simulink model "mpc_tgt_calc"  (R2020a)
settings: Solver=ode1  StartTime=0.0  StopTime=2600  FixedStep=0.1  RelTol=1e-3
undefined symbols (not defined in the file): accl, alpha, ang, dist, dt, ideal_point, img_ang, img_dist, kanayama_point, pivot_state, sla_param, slip_point, state, trj_diff, v, w
libraries: simulink x1
settings Model: Creator=nao12  LastModifiedBy=nao12
settings DataIOCC: SaveOutput=off  SignalLogging=off  DSMLogging=off  SaveTime=off  ReturnWorkspaceOutputs=off
settings OptimizationCC: EnhancedBackFolding=on  PassReuseOutputArgsAs=Individual arguments  OptimizeBlockOrder=speed  DifferentSizesBufferReuse=on  OptimizationCustomize=off  EfficientTunableParamExpr=on
settings DebuggingCC: ParameterTunabilityLossMsg=error  ArithmeticOperatorsInVariantConditions=warning
settings SFSimCC: SimCustomHeaderCode="#include \"bus.h\""  SimUserIncludeDirs=../include/  MATLABDynamicMemAlloc=off  CustomCodeUndefinedFunction=UseInterfaceOnly
settings RTWCC: SystemTargetFile=ert.tlc  GenCodeOnly=on  TemplateMakefile=ert_default_tmf  GenerateReport=on  RTWUseSimCustomCode=on  CustomHeaderCode="#include \"bus.h\""  CustomInclude=../include/  IncludeHyperlinkInReport=on  LaunchReport=on  GenerateTraceInfo=on  GenerateTraceReport=on  GenerateTraceReportSl=on  GenerateTraceReportSf=on  GenerateTraceReportEml=on
settings CodeAppCC: GenerateComments=off  IgnoreCustomStorageClasses=off  OperatorAnnotations=on  SimulinkDataObjDesc=on  SFDataObjDesc=on  InsertBlockDesc=on
settings ERTTargetCC: TargetLangStandard=C99 (ISO)  GenerateSampleERTMain=on  SupportAbsoluteTime=off  MultiInstanceERTCode=on  CodeInterfacePackaging=Reusable function  SupportComplex=off  ParenthesesLevel=Minimum  ERTCustomFileTemplate=example_file_process.tlc  EnableUserReplacementTypes=on

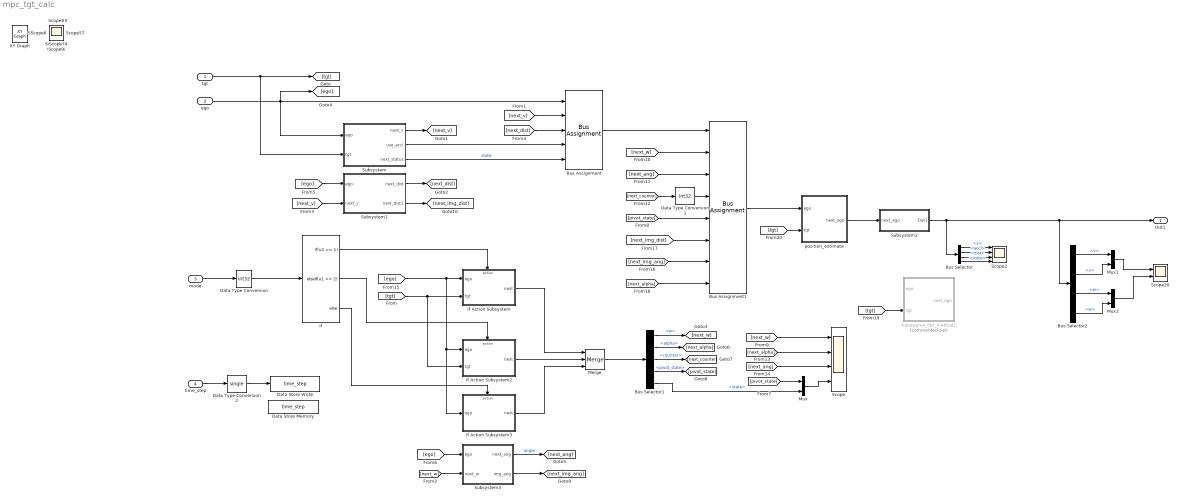
== system mpc_tgt_calc ==
  tgt : Inport  OutDataTypeStr=Bus: t_tgt  BusOutputAsStruct=on
  ego : Inport  Port=2  OutDataTypeStr=Bus: t_ego  BusOutputAsStruct=on
  mode : Inport  Port=3  OutDataTypeStr=int32
  time_step : Inport  Port=4  OutDataTypeStr=int32
  Bus Assignment : BusAssignment  AssignedSignals=v,dist,accl,state
  Bus Assignment1 : BusAssignment  AssignedSignals=w,ang,sla_param.counter,pivot_state,img_dist,img_ang,alpha
  Bus Selector : BusSelector  OutputSignals=v,accl,dist,state
  Bus Selector1 : BusSelector  OutputSignals=w,alpha,sla_param.counter,pivot_state,sla_param.state
  Bus Selector2 : BusSelector  OutputSignals=v,kanayama_point.v,w,kanayama_point.w
  Data Store Memory : DataStoreMemory  DataStoreName=time_step  ReadBeforeWriteMsg=warning  WriteAfterWriteMsg=warning  WriteAfterReadMsg=warning  ShowAdditionalParam=off
  Data Store Write : DataStoreWrite  DataStoreName=time_step
  Data Type Conversion : DataTypeConversion  OutDataTypeStr=int32
  Data Type Conversion1 : DataTypeConversion  OutDataTypeStr=int32
  Data Type Conversion2 : DataTypeConversion  OutDataTypeStr=single
  If : If  IfExpression=u1 == 1  ElseIfExpressions=u1 == 2
  If Action Subsystem : Subsystem  TreatAsAtomicUnit=on
  If Action Subsystem2 : Subsystem  TreatAsAtomicUnit=on
  If Action Subsystem3 : Subsystem  TreatAsAtomicUnit=on
  Merge : Merge  Inputs=3
  Mux : Mux  Inputs=2
  Mux1 : Mux  Inputs=2
  Mux2 : Mux  Inputs=2
  Scope : Scope  NumInputPorts=4
  Scope2 : Scope  NumInputPorts=4
  Scope20 : Scope  NumInputPorts=2
  Subsystem : Subsystem
  Subsystem1 : Subsystem
  Subsystem2 : Subsystem
  Subsystem3 : Subsystem
  kanayama_ctrl_method1 : Subsystem  Commented=on
  position_estimate : Subsystem
  Out1 : Outport  OutDataTypeStr=Bus: t_ego
  Scope{1,3..19} (18 alike) : Scope
  XY Graph : simulink/Sinks/XY Graph  IOType=viewer  xmin=-1  xmax=1  ymin=-1  ymax=1  st=-1
  wires:
  mode/1 -> Data Type Conversion/1
  tgt/1 -> [tgt], Subsystem/2(tgt)
  ego/1 -> Subsystem/1(ego), Bus Assignment/1, [ego]
  Data Type Conversion/1 -> If/1
  If/1 -> If Action Subsystem/Action
  [tgt] -> If Action Subsystem2/2(tgt), If Action Subsystem/2(tgt)
  Bus Assignment/1 -> Bus Assignment1/1
  [next_v] -> Bus Assignment/2
  [next_dist] -> Bus Assignment/3
  Subsystem/1(next_v) -> [next_v]
  [next_v] -> Subsystem1/2(next_v)
  Subsystem1/1(next_dist) -> [next_dist]
  Subsystem/2(use_accl) -> Bus Assignment/4
  Subsystem/3(next_status) -> Bus Assignment/5  "state"
  [next_w] -> Subsystem3/2(next_w)
  [ego] -> Subsystem1/1(ego)
  [ego] -> Subsystem3/1(ego)
  Subsystem3/1(next_ang) -> [next_ang]  "angle"
  Bus Selector/4 -> Scope2/4  "<state>"
  Bus Selector/1 -> Scope2/1  "<v>"
  Bus Selector/2 -> Scope2/2  "<accl>"
  Bus Selector/3 -> Scope2/3  "<dist>"
  Bus Assignment1/1 -> position_estimate/1(ego)
  [next_w] -> Bus Assignment1/2
  [next_ang] -> Bus Assignment1/3
  [next_counter] -> Data Type Conversion1/1
  Data Type Conversion1/1 -> Bus Assignment1/4
  [next_w] -> Scope/1
  [next_alpha] -> Scope/2
  [next_ang] -> Scope/3
  If/2 -> If Action Subsystem2/Action
  [ego] -> If Action Subsystem3/1(ego), If Action Subsystem2/1(ego), If Action Subsystem/1(ego)
  If/3 -> If Action Subsystem3/Action
  Merge/1 -> Bus Selector1/1
  Bus Selector1/1 -> [next_w]  "<w>"
  Bus Selector1/2 -> [next_alpha]  "<alpha>"
  Bus Selector1/3 -> [next_counter]  "<counter>"
  If Action Subsystem/1(next) -> Merge/1
  If Action Subsystem2/1(next) -> Merge/2
  If Action Subsystem3/1(next) -> Merge/3
  Bus Selector1/4 -> [pivot_state]  "<pivot_state>"
  [pivot_state] -> Bus Assignment1/5
  Mux/1 -> Scope/4
  [pivot_state] -> Mux/1
  Bus Selector1/5 -> Mux/2  "<state>"
  Subsystem3/2(img_ang) -> [next_img_ang]
  [next_img_ang] -> Bus Assignment1/7
  Subsystem1/2(next_dist1) -> [next_img_dist]
  [next_img_dist] -> Bus Assignment1/6
  position_estimate/1(next_ego) -> Subsystem2/1(next_ego)
  [next_alpha] -> Bus Assignment1/8
  Subsystem2/1(Out1) -> Bus Selector/1, Out1/1, Bus Selector2/1
  [tgt] -> kanayama_ctrl_method1/2(tgt)
  Mux1/1 -> Scope20/1
  Bus Selector2/1 -> Mux1/1  "<v>"
  Mux2/1 -> Scope20/2
  Bus Selector2/2 -> Mux1/2  "<v>"
  Bus Selector2/3 -> Mux2/1  "<w>"
  Bus Selector2/4 -> Mux2/2  "<w>"
  [tgt] -> position_estimate/2(tgt)
  time_step/1 -> Data Type Conversion2/1
  Data Type Conversion2/1 -> Data Store Write/1

== system mpc_tgt_calc/If Action Subsystem ==
  ego : Inport
  tgt : Inport  Port=2
  Action Port : ActionPort  ActionPortLabel=if(u1 == 1)
  Bus Assignment : BusAssignment  AssignedSignals=w,alpha,sla_param.counter
  Data Type Conversion : DataTypeConversion  OutDataTypeStr=int32
  Data Type Conversion1 : DataTypeConversion  OutDataTypeStr=single
  Data Type Conversion2 : DataTypeConversion  OutDataTypeStr=single
  Subsystem2 : Subsystem
  next : Outport
  wires:
  ego/1 -> Subsystem2/1(ego), Bus Assignment/1
  tgt/1 -> Subsystem2/2(tgt)
  Bus Assignment/1 -> next/1
  Subsystem2/1(next_w) -> Data Type Conversion1/1
  Subsystem2/2(next_alpha) -> Data Type Conversion2/1
  Subsystem2/3(next_count) -> Data Type Conversion/1
  Data Type Conversion/1 -> Bus Assignment/4
  Data Type Conversion1/1 -> Bus Assignment/2
  Data Type Conversion2/1 -> Bus Assignment/3

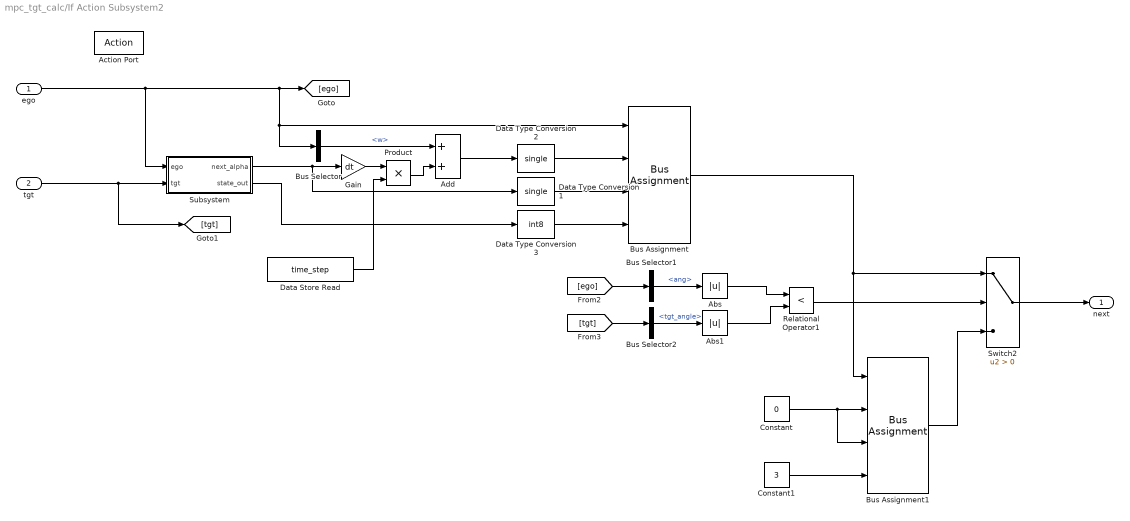
== system mpc_tgt_calc/If Action Subsystem2 ==
  ego : Inport
  tgt : Inport  Port=2
  Action Port : ActionPort  ActionPortLabel=elseif(u1 == 2)
  Abs : Abs
  Abs1 : Abs
  Add : Sum
  Bus Assignment : BusAssignment  AssignedSignals=w,alpha,pivot_state
  Bus Assignment1 : BusAssignment  AssignedSignals=w,alpha,pivot_state
  Bus Selector : BusSelector  OutputSignals=w
  Bus Selector1 : BusSelector  OutputSignals=ang
  Bus Selector2 : BusSelector  OutputSignals=tgt_angle
  Constant : Constant  Value=0  OutDataTypeStr=single
  Constant1 : Constant  Value=3  OutDataTypeStr=int8
  Data Store Read : DataStoreRead  DataStoreName=time_step
  Data Type Conversion1 : DataTypeConversion  OutDataTypeStr=single
  Data Type Conversion2 : DataTypeConversion  OutDataTypeStr=single
  Data Type Conversion3 : DataTypeConversion  OutDataTypeStr=int8
  Gain : Gain  Gain=dt
  Product : Product
  Relational Operator1 : RelationalOperator  Operator=<  OutDataTypeStr=boolean  RndMeth=Simplest
  Subsystem : Subsystem
  Switch2 : Switch  Criteria=u2 > Threshold
  next : Outport
  wires:
  ego/1 -> Subsystem/1(ego), Bus Selector/1, Bus Assignment/1, [ego]
  Subsystem/1(next_alpha) -> Data Type Conversion1/1, Gain/1
  Bus Selector/1 -> Add/1  "<w>"
  Add/1 -> Data Type Conversion2/1
  Data Type Conversion2/1 -> Bus Assignment/2
  tgt/1 -> [tgt], Subsystem/2(tgt)
  Data Type Conversion1/1 -> Bus Assignment/3
  Data Type Conversion3/1 -> Bus Assignment/4
  Subsystem/2(state_out) -> Data Type Conversion3/1
  Bus Assignment/1 -> Bus Assignment1/1, Switch2/1
  Relational Operator1/1 -> Switch2/2
  Bus Selector2/1 -> Abs1/1  "<tgt_angle>"
  Abs/1 -> Relational Operator1/1
  [ego] -> Bus Selector1/1
  [tgt] -> Bus Selector2/1
  Bus Selector1/1 -> Abs/1  "<ang>"
  Abs1/1 -> Relational Operator1/2
  Switch2/1 -> next/1
  Constant/1 -> Bus Assignment1/3, Bus Assignment1/2
  Constant1/1 -> Bus Assignment1/4
  Bus Assignment1/1 -> Switch2/3
  Data Store Read/1 -> Product/2
  Gain/1 -> Product/1
  Product/1 -> Add/2

== system mpc_tgt_calc/If Action Subsystem3 ==
  ego : Inport
  Action Port : ActionPort  ActionPortLabel=else
  next : Outport
  wires:
  ego/1 -> next/1

== system mpc_tgt_calc/Subsystem ==
  ego : Inport
  tgt : Inport  Port=2
  Bus Selector2 : BusSelector  OutputSignals=v_max
  If : If  IfExpression=u1 >= 0
  Merge : Merge
  Merge1 : Merge
  Merge2 : Merge
  straight_ahead : Subsystem  TreatAsAtomicUnit=on
  straight_back : Subsystem  TreatAsAtomicUnit=on
  next_v : Outport
  use_accl : Outport  Port=2
  next_status : Outport  Port=3
  wires:
  tgt/1 -> [tgt], Bus Selector2/1
  Bus Selector2/1 -> If/1  "<v_max>"
  If/1 -> straight_ahead/Action
  ego/1 -> [ego]
  [ego] -> straight_ahead/1(ego)
  [tgt] -> straight_ahead/2(tgt)
  [ego] -> straight_back/1(ego)
  [tgt] -> straight_back/2(tgt)
  If/2 -> straight_back/Action
  straight_ahead/1(next_v) -> Merge/1
  straight_ahead/2(use_accl) -> Merge1/1
  straight_ahead/3(next_status) -> Merge2/1
  straight_back/1(next_v) -> Merge/2
  straight_back/2(use_accl) -> Merge1/2
  straight_back/3(next_status) -> Merge2/2
  Merge/1 -> next_v/1
  Merge1/1 -> use_accl/1
  Merge2/1 -> next_status/1

== system mpc_tgt_calc/Subsystem1 ==
  ego : Inport
  next_v : Inport  Port=2
  Add1 : Sum
  Add2 : Sum
  Bus Selector : BusSelector  OutputSignals=dist,img_dist
  Data Store Read : DataStoreRead  DataStoreName=time_step
  Data Type Conversion1 : DataTypeConversion  OutDataTypeStr=single
  Data Type Conversion2 : DataTypeConversion  OutDataTypeStr=single
  Gain1 : Gain  Gain=dt
  Product : Product
  next_dist : Outport
  next_dist1 : Outport  Port=2
  wires:
  ego/1 -> Bus Selector/1
  Bus Selector/1 -> Add1/1  "<dist>"
  Add1/1 -> Data Type Conversion1/1
  Data Type Conversion1/1 -> next_dist/1
  Add2/1 -> Data Type Conversion2/1
  Gain1/1 -> Add2/2, Add1/2
  Data Type Conversion2/1 -> next_dist1/1
  Bus Selector/2 -> Add2/1  "<img_dist>"
  Product/1 -> Gain1/1
  next_v/1 -> Product/1
  Data Store Read/1 -> Product/2

== system mpc_tgt_calc/Subsystem2 ==
  next_ego : Inport
  Out1 : Outport
  wires:
  next_ego/1 -> Out1/1

== system mpc_tgt_calc/Subsystem3 ==
  ego : Inport
  next_w : Inport  Port=2
  Add1 : Sum
  Add2 : Sum
  Bus Selector : BusSelector  OutputSignals=ang,img_ang
  Data Store Read : DataStoreRead  DataStoreName=time_step
  Data Type Conversion1 : DataTypeConversion  OutDataTypeStr=single
  Data Type Conversion2 : DataTypeConversion  OutDataTypeStr=single
  Gain1 : Gain  Gain=dt
  Product : Product
  next_ang : Outport
  img_ang : Outport  Port=2
  wires:
  ego/1 -> Bus Selector/1
  Add1/1 -> Data Type Conversion1/1
  Bus Selector/1 -> Add1/1  "<ang>"
  Data Type Conversion1/1 -> next_ang/1
  Bus Selector/2 -> Add2/1  "<img_ang>"
  Data Type Conversion2/1 -> img_ang/1
  Add2/1 -> Data Type Conversion2/1
  Gain1/1 -> Add1/2, Add2/2
  Data Store Read/1 -> Product/2
  Product/1 -> Gain1/1
  next_w/1 -> Product/1

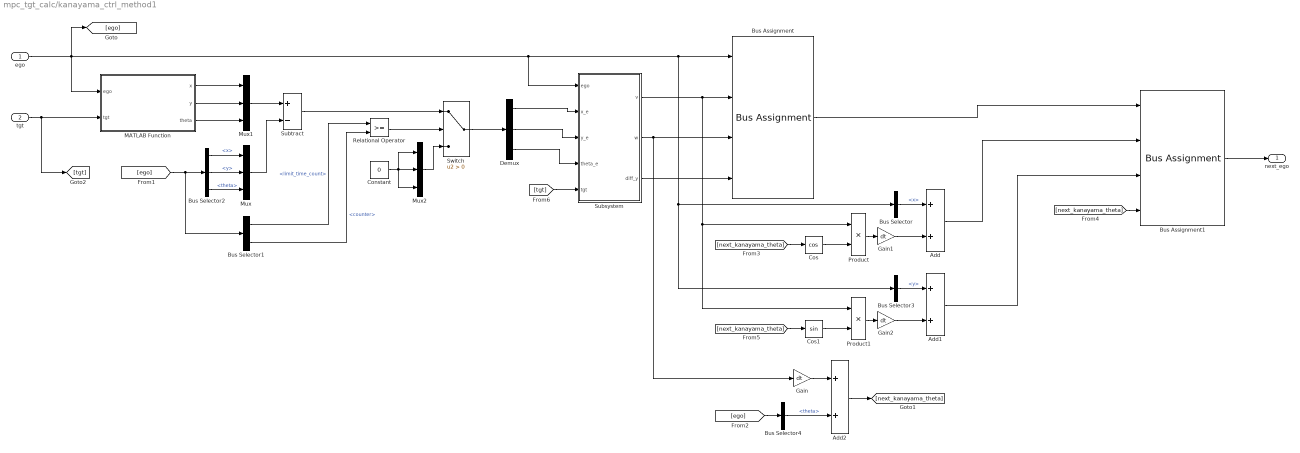
== system mpc_tgt_calc/kanayama_ctrl_method1 ==
  ego : Inport
  tgt : Inport  Port=2
  Add : Sum
  Add1 : Sum
  Add2 : Sum
  Bus Assignment : BusAssignment  AssignedSignals=kanayama_point.v,kanayama_point.w,kanayama_point.diff_y
  Bus Assignment1 : BusAssignment  AssignedSignals=kanayama_point.x,kanayama_point.y,kanayama_point.theta
  Bus Selector : BusSelector  OutputSignals=kanayama_point.x
  Bus Selector1 : BusSelector  OutputSignals=sla_param.limit_time_count,sla_param.counter
  Bus Selector2 : BusSelector  OutputSignals=slip_point.x,slip_point.y,slip_point.theta
  Bus Selector3 : BusSelector  OutputSignals=kanayama_point.y
  Bus Selector4 : BusSelector  OutputSignals=kanayama_point.theta
  Constant : Constant  Value=0  OutDataTypeStr=single
  Cos : Trigonometry  Operator=cos
  Cos1 : Trigonometry
  Demux : Demux  Outputs=3
  Gain : Gain  Gain=dt
  Gain1 : Gain  Gain=dt
  Gain2 : Gain  Gain=dt
  MATLAB Function : MATLAB Function  TreatAsAtomicUnit=on
  Mux : Mux  Inputs=3
  Mux1 : Mux  Inputs=3
  Mux2 : Mux  Inputs=3
  Product : Product
  Product1 : Product
  Relational Operator : RelationalOperator  OutDataTypeStr=boolean  RndMeth=Simplest
  Subsystem : Subsystem
  Subtract : Sum  Inputs=+-
  Switch : Switch  Criteria=u2 > Threshold
  next_ego : Outport
  wires:
  tgt/1 -> [tgt], MATLAB Function/2(tgt)
  Bus Selector2/1 -> Mux/1  "<x>"
  Bus Selector2/2 -> Mux/2  "<y>"
  Bus Selector2/3 -> Mux/3  "<theta>"
  MATLAB Function/1(x) -> Mux1/1
  MATLAB Function/2(y) -> Mux1/2
  MATLAB Function/3(theta) -> Mux1/3
  Mux1/1 -> Subtract/1
  Mux/1 -> Subtract/2
  Switch/1 -> Demux/1
  Bus Selector1/1 -> Relational Operator/1  "<limit_time_count>"
  Bus Selector1/2 -> Relational Operator/2  "<counter>"
  Relational Operator/1 -> Switch/2
  Subtract/1 -> Switch/1
  Mux2/1 -> Switch/3
  Constant/1 -> Mux2/1, Mux2/2, Mux2/3
  Bus Assignment/1 -> Bus Assignment1/1
  Demux/1 -> Subsystem/2(x_e)
  Demux/2 -> Subsystem/3(y_e)
  Demux/3 -> Subsystem/4(theta_e)
  Subsystem/2(w) -> Gain/1, Bus Assignment/3
  Product/1 -> Gain1/1
  Bus Selector/1 -> Add/1  "<x>"
  Add/1 -> Bus Assignment1/2
  Add1/1 -> Bus Assignment1/3
  Cos/1 -> Product/2
  Subsystem/1(v) -> Product/1, Product1/1, Bus Assignment/2
  [next_kanayama_theta] -> Cos/1
  Gain1/1 -> Add/2
  Cos1/1 -> Product1/2
  Gain2/1 -> Add1/2
  ego/1 -> MATLAB Function/1(ego), [ego], Subsystem/1(ego), Bus Selector3/1, Bus Selector/1, Bus Assignment/1
  Product1/1 -> Gain2/1
  Bus Assignment1/1 -> next_ego/1
  [ego] -> Bus Selector1/1, Bus Selector2/1
  [ego] -> Bus Selector4/1
  Gain/1 -> Add2/1
  Bus Selector4/1 -> Add2/2  "<theta>"
  Add2/1 -> [next_kanayama_theta]
  Bus Selector3/1 -> Add1/1  "<y>"
  [next_kanayama_theta] -> Bus Assignment1/4
  [next_kanayama_theta] -> Cos1/1
  [tgt] -> Subsystem/5(tgt)
  Subsystem/3(diff_y) -> Bus Assignment/4

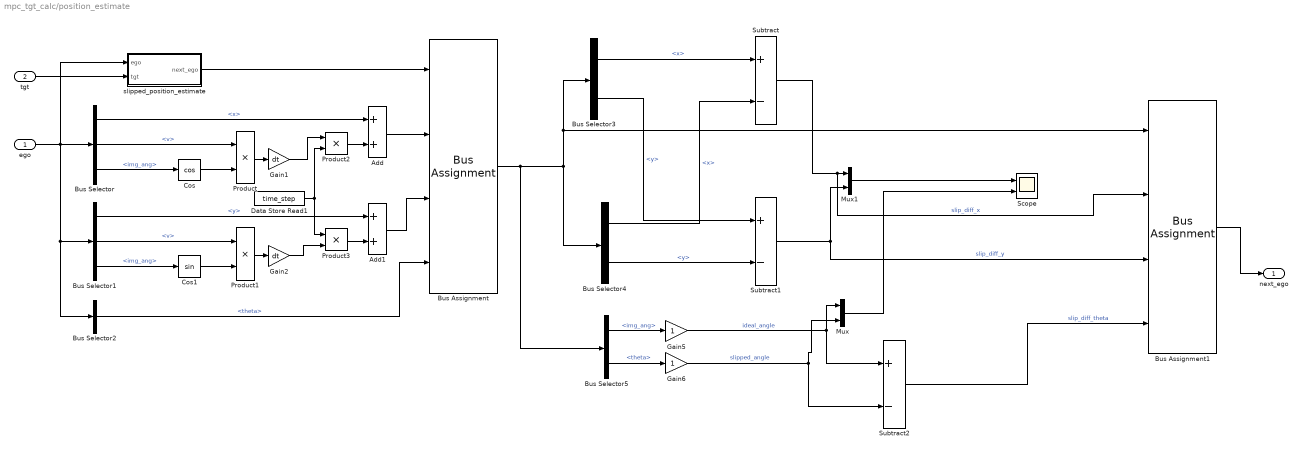
== system mpc_tgt_calc/position_estimate ==
  ego : Inport
  tgt : Inport  Port=2
  Add : Sum
  Add1 : Sum
  Bus Assignment : BusAssignment  AssignedSignals=ideal_point.x,ideal_point.y,ideal_point.theta
  Bus Assignment1 : BusAssignment  AssignedSignals=trj_diff.x,trj_diff.y,trj_diff.theta
  Bus Selector : BusSelector  OutputSignals=ideal_point.x,v,img_ang
  Bus Selector1 : BusSelector  OutputSignals=ideal_point.y,v,img_ang
  Bus Selector2 : BusSelector  OutputSignals=ideal_point.theta
  Bus Selector3 : BusSelector  OutputSignals=ideal_point.x,ideal_point.y
  Bus Selector4 : BusSelector  OutputSignals=slip_point.x,slip_point.y
  Bus Selector5 : BusSelector  OutputSignals=img_ang,slip_point.theta
  Cos : Trigonometry  Operator=cos
  Cos1 : Trigonometry
  Data Store Read1 : DataStoreRead  DataStoreName=time_step
  Gain1 : Gain  Gain=dt
  Gain2 : Gain  Gain=dt
  Gain5 : Gain
  Gain6 : Gain
  Mux : Mux  Inputs=2
  Mux1 : Mux  Inputs=2
  Product{,1..3} (4 alike) : Product
  Scope : Scope  NumInputPorts=2
  Subtract : Sum  Inputs=+-
  Subtract1 : Sum  Inputs=+-
  Subtract2 : Sum  Inputs=+-
  slipped_position_estimate : Subsystem
  next_ego : Outport
  wires:
  ego/1 -> slipped_position_estimate/1(ego), Bus Selector1/1, Bus Selector2/1, Bus Selector/1
  Bus Selector/1 -> Add/1  "<x>"
  Bus Selector/2 -> Product/1  "<v>"
  Bus Selector/3 -> Cos/1  "<img_ang>"
  Cos/1 -> Product/2
  Product/1 -> Gain1/1
  Bus Selector1/2 -> Product1/1  "<v>"
  Bus Selector1/1 -> Add1/1  "<y>"
  Product1/1 -> Gain2/1
  Bus Selector1/3 -> Cos1/1  "<img_ang>"
  Cos1/1 -> Product1/2
  Bus Selector2/1 -> Bus Assignment/4  "<theta>"
  Add1/1 -> Bus Assignment/3
  Add/1 -> Bus Assignment/2
  Bus Selector3/1 -> Subtract/1  "<x>"
  Bus Selector3/2 -> Subtract1/1  "<y>"
  slipped_position_estimate/1(next_ego) -> Bus Assignment/1
  Bus Selector4/1 -> Subtract/2  "<x>"
  Bus Selector4/2 -> Subtract1/2  "<y>"
  Subtract/1 -> Bus Assignment1/2, Mux1/1  "slip_diff_x"
  Subtract1/1 -> Mux1/2, Bus Assignment1/3  "slip_diff_y"
  Bus Assignment/1 -> Bus Selector5/1, Bus Selector3/1, Bus Assignment1/1, Bus Selector4/1
  Bus Selector5/2 -> Gain6/1  "<theta>"
  Gain6/1 -> Mux/2, Subtract2/2  "slipped_angle"
  Gain5/1 -> Mux/1, Subtract2/1  "ideal_angle"
  Bus Selector5/1 -> Gain5/1  "<img_ang>"
  Mux/1 -> Scope/2
  Mux1/1 -> Scope/1
  Bus Assignment1/1 -> next_ego/1
  Subtract2/1 -> Bus Assignment1/4  "slip_diff_theta"
  tgt/1 -> slipped_position_estimate/2(tgt)
  Product2/1 -> Add/2
  Gain1/1 -> Product2/1
  Product3/1 -> Add1/2
  Data Store Read1/1 -> Product3/1, Product2/2
  Gain2/1 -> Product3/2

== system mpc_tgt_calc/If Action Subsystem/Subsystem2 ==
  ego : Inport
  tgt : Inport  Port=2
  Add : Sum
  Add1 : Sum
  Bus Selector : BusSelector  OutputSignals=w,sla_param,sla_param.counter
  Bus Selector1 : BusSelector  OutputSignals=sla_param.counter,sla_param.limit_time_count
  Constant1 : Constant  Value=0
  Data Store Read : DataStoreRead  DataStoreName=time_step
  Data Store Read1 : DataStoreRead  DataStoreName=time_step
  Data Type Conversion : DataTypeConversion  OutDataTypeStr=single
  Data Type Conversion1 : DataTypeConversion  OutDataTypeStr=single
  Data Type Conversion2 : DataTypeConversion  OutDataTypeStr=single
  Gain : Gain  Gain=dt
  Product : Product
  Relational Operator : RelationalOperator  OutDataTypeStr=boolean  RndMeth=Simplest
  Scope : Scope  NumInputPorts=3
  Subsystem : Subsystem
  Switch : Switch  Criteria=u2 > Threshold
  Terminator : Terminator
  next_w : Outport
  next_alpha : Outport  Port=2
  next_count : Outport  Port=3
  wires:
  Bus Selector/1 -> Add/1  "<w>"
  Subsystem/1(next_alpha) -> Gain/1, Scope/2, next_alpha/1
  Bus Selector/2 -> Subsystem/1(ego)  "<sla_param>"
  Bus Selector/3 -> Add1/1  "<counter>"
  Data Store Read1/1 -> Data Type Conversion2/1
  Add1/1 -> Data Type Conversion1/1
  Data Type Conversion/1 -> Add/2
  Data Type Conversion2/1 -> Add1/2
  Data Type Conversion1/1 -> Scope/3, next_count/1
  tgt/1 -> Terminator/1
  Bus Selector1/2 -> Relational Operator/2  "<limit_time_count>"
  Relational Operator/1 -> Switch/2
  ego/1 -> Bus Selector1/1, Bus Selector/1
  Bus Selector1/1 -> Relational Operator/1  "<counter>"
  Constant1/1 -> Switch/1
  Add/1 -> Switch/3
  Switch/1 -> Scope/1, next_w/1
  Data Store Read/1 -> Product/1
  Gain/1 -> Product/2
  Product/1 -> Data Type Conversion/1

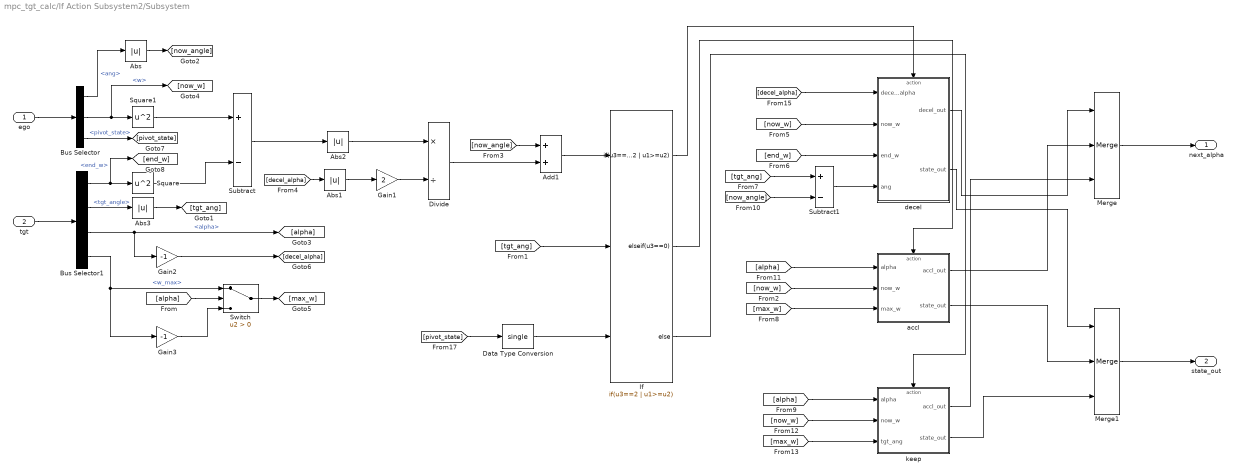
== system mpc_tgt_calc/If Action Subsystem2/Subsystem ==
  ego : Inport
  tgt : Inport  Port=2
  Abs{,1..3} (4 alike) : Abs
  Add1 : Sum
  Bus Selector : BusSelector  OutputSignals=ang,w,pivot_state
  Bus Selector1 : BusSelector  OutputSignals=end_w,tgt_angle,alpha,w_max
  Data Type Conversion : DataTypeConversion  OutDataTypeStr=single
  Divide : Product  Inputs=*/
  Gain1 : Gain  Gain=2
  Gain2 : Gain  Gain=-1
  Gain3 : Gain  Gain=-1
  If : If  NumInputs=3  IfExpression=u3==2 | u1>=u2  ElseIfExpressions=u3==0
  Merge : Merge  Inputs=3
  Merge1 : Merge  Inputs=3
  Square : Math  Operator=square  SaturateOnIntegerOverflow=on
  Square1 : Math  Operator=square  SaturateOnIntegerOverflow=on
  Subtract : Sum  Inputs=+-
  Subtract1 : Sum  Inputs=+-
  Switch : Switch  Criteria=u2 > Threshold
  accl : Subsystem  TreatAsAtomicUnit=on
  decel : Subsystem  TreatAsAtomicUnit=on
  keep : Subsystem  TreatAsAtomicUnit=on
  next_alpha : Outport
  state_out : Outport  Port=2
  wires:
  ego/1 -> Bus Selector/1
  Subtract/1 -> Abs2/1
  Divide/1 -> Add1/2
  [now_angle] -> Add1/1
  Abs1/1 -> Gain1/1
  Abs2/1 -> Divide/1
  [decel_alpha] -> Abs1/1
  Gain1/1 -> Divide/2
  tgt/1 -> Bus Selector1/1
  Bus Selector1/1 -> [end_w], Square/1  "<end_w>"
  Square/1 -> Subtract/2
  Square1/1 -> Subtract/1
  Bus Selector/3 -> [pivot_state]  "<pivot_state>"
  Bus Selector/2 -> [now_w], Square1/1  "<w>"
  Bus Selector/1 -> Abs/1  "<ang>"
  Bus Selector1/2 -> Abs3/1  "<tgt_angle>"
  Bus Selector1/3 -> Gain2/1, [alpha]  "<alpha>"
  Gain2/1 -> [decel_alpha]
  Switch/1 -> [max_w]
  [alpha] -> Switch/2
  Bus Selector1/4 -> Gain3/1, Switch/1  "<w_max>"
  Gain3/1 -> Switch/3
  [pivot_state] -> Data Type Conversion/1
  Data Type Conversion/1 -> If/3
  [tgt_ang] -> If/2
  Add1/1 -> If/1
  keep/2(state_out) -> Merge1/3
  decel/1(decel_out) -> Merge/1
  [max_w] -> keep/3(tgt_ang)
  accl/1(accl_out) -> Merge/2
  [now_w] -> keep/2(now_w)
  [decel_alpha] -> decel/1(decel_alpha)
  [now_w] -> decel/2(now_w)
  [now_angle] -> Subtract1/2
  [tgt_ang] -> Subtract1/1
  [now_w] -> accl/2(now_w)
  accl/2(state_out) -> Merge1/2
  If/2 -> accl/Action
  keep/1(accl_out) -> Merge/3
  [max_w] -> accl/3(max_w)
  [alpha] -> keep/1(alpha)
  If/3 -> keep/Action
  [end_w] -> decel/3(end_w)
  decel/2(state_out) -> Merge1/1
  Merge1/1 -> state_out/1
  Subtract1/1 -> decel/4(ang)
  If/1 -> decel/Action
  Merge/1 -> next_alpha/1
  [alpha] -> accl/1(alpha)
  Abs/1 -> [now_angle]
  Abs3/1 -> [tgt_ang]

== system mpc_tgt_calc/Subsystem/straight_ahead ==
  ego : Inport
  tgt : Inport  Port=2
  Action Port : ActionPort  ActionPortLabel=if(u1 >= 0)
  Add : Sum
  Bus Selector : BusSelector  OutputSignals=v
  Bus Selector1 : BusSelector  OutputSignals=v_max
  Constant : Constant  Value=0  OutDataTypeStr=single
  Data Store Read : DataStoreRead  DataStoreName=time_step
  Data Type Conversion2 : DataTypeConversion  OutDataTypeStr=single
  Gain : Gain  Gain=dt
  Max : MinMax  Function=max  Inputs=2
  Min : MinMax  Inputs=2
  Product : Product
  Subsystem : Subsystem
  next_v : Outport
  use_accl : Outport  Port=2
  next_status : Outport  Port=3
  wires:
  Max/1 -> next_v/1
  Subsystem/1(use_accl) -> use_accl/1, Gain/1
  Constant/1 -> Max/2
  Bus Selector/1 -> Add/1  "<v>"
  ego/1 -> Subsystem/1(ego), Bus Selector/1
  tgt/1 -> Subsystem/2(tgt), Bus Selector1/1
  Data Type Conversion2/1 -> Min/2
  Min/1 -> Max/1  "velocity"
  Bus Selector1/1 -> Min/1  "<v_max>"
  Subsystem/2(next_state) -> next_status/1
  Add/1 -> Data Type Conversion2/1
  Data Store Read/1 -> Product/1
  Product/1 -> Add/2
  Gain/1 -> Product/2

== system mpc_tgt_calc/Subsystem/straight_back ==
  ego : Inport
  tgt : Inport  Port=2
  Action Port : ActionPort  ActionPortLabel=else
  Add : Sum
  Bus Selector : BusSelector  OutputSignals=v
  Bus Selector1 : BusSelector  OutputSignals=v_max
  Constant : Constant  Value=0  OutDataTypeStr=single
  Data Store Read : DataStoreRead  DataStoreName=time_step
  Data Type Conversion2 : DataTypeConversion  OutDataTypeStr=single
  Gain : Gain  Gain=dt
  Max : MinMax  Inputs=2
  Min : MinMax  Function=max  Inputs=2
  Product : Product
  Subsystem : Subsystem
  next_v : Outport
  use_accl : Outport  Port=2
  next_status : Outport  Port=3
  wires:
  Max/1 -> next_v/1
  Subsystem/1(use_accl) -> use_accl/1, Gain/1
  Constant/1 -> Max/2
  Bus Selector/1 -> Add/1  "<v>"
  ego/1 -> Subsystem/1(ego), Bus Selector/1
  tgt/1 -> Subsystem/2(tgt), Bus Selector1/1
  Data Type Conversion2/1 -> Min/2
  Min/1 -> Max/1  "velocity"
  Bus Selector1/1 -> Min/1  "<v_max>"
  Subsystem/2(next_state) -> next_status/1
  Add/1 -> Data Type Conversion2/1
  Data Store Read/1 -> Product/1
  Product/1 -> Add/2
  Gain/1 -> Product/2

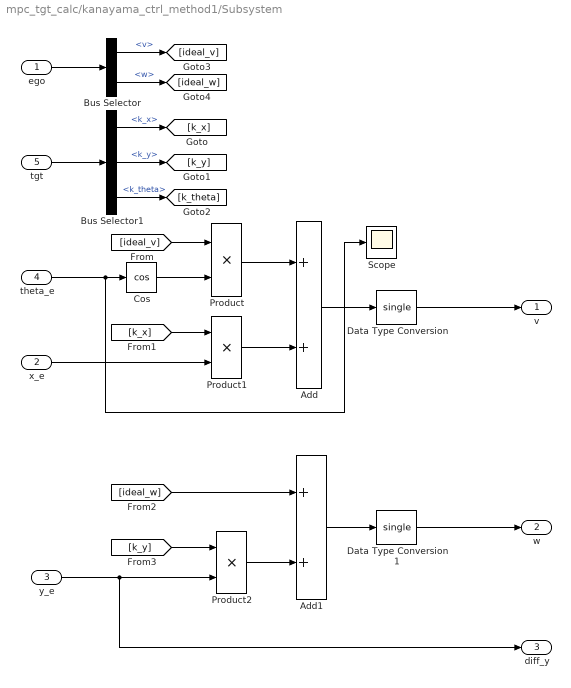
== system mpc_tgt_calc/kanayama_ctrl_method1/Subsystem ==
  ego : Inport
  x_e : Inport  Port=2
  y_e : Inport  Port=3
  theta_e : Inport  Port=4
  tgt : Inport  Port=5
  Add : Sum
  Add1 : Sum
  Bus Selector : BusSelector  OutputSignals=v,w
  Bus Selector1 : BusSelector  OutputSignals=kanayama_gain.k_x,kanayama_gain.k_y,kanayama_gain.k_theta
  Cos : Trigonometry  Operator=cos
  Data Type Conversion : DataTypeConversion  OutDataTypeStr=single
  Data Type Conversion1 : DataTypeConversion  OutDataTypeStr=single
  Product : Product
  Product1 : Product
  Product2 : Product
  Scope : Scope
  v : Outport
  w : Outport  Port=2
  diff_y : Outport  Port=3
  wires:
  ego/1 -> Bus Selector/1
  tgt/1 -> Bus Selector1/1
  Bus Selector1/1 -> [k_x]  "<k_x>"
  Bus Selector1/2 -> [k_y]  "<k_y>"
  Bus Selector1/3 -> [k_theta]  "<k_theta>"
  Bus Selector/1 -> [ideal_v]  "<v>"
  Bus Selector/2 -> [ideal_w]  "<w>"
  [ideal_v] -> Product/1
  Cos/1 -> Product/2
  Product/1 -> Add/1
  Product1/1 -> Add/2
  [k_x] -> Product1/1
  [ideal_w] -> Add1/1
  Add/1 -> Data Type Conversion/1
  Data Type Conversion/1 -> v/1
  theta_e/1 -> Scope/1, Cos/1
  Add1/1 -> Data Type Conversion1/1
  Data Type Conversion1/1 -> w/1
  x_e/1 -> Product1/2
  Product2/1 -> Add1/2
  y_e/1 -> diff_y/1, Product2/2
  [k_y] -> Product2/1

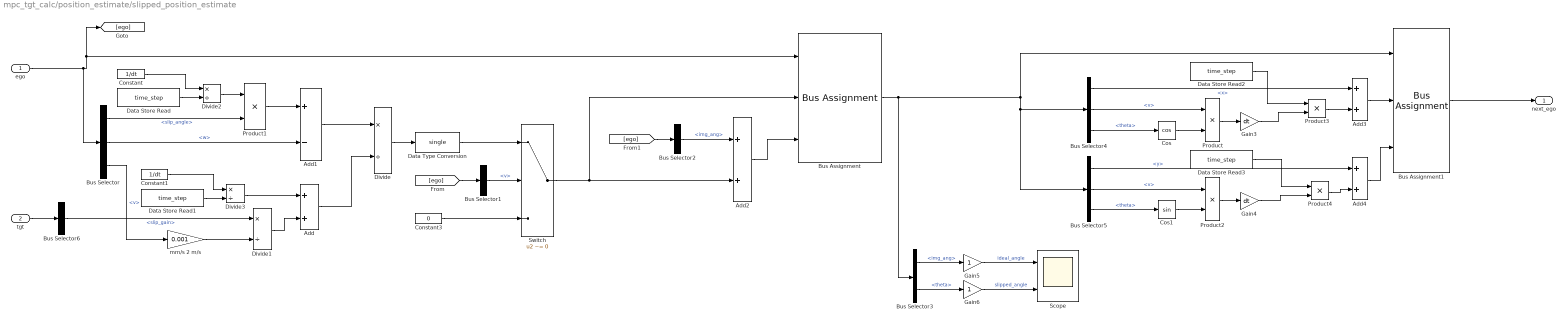
== system mpc_tgt_calc/position_estimate/slipped_position_estimate ==
  ego : Inport
  tgt : Inport  Port=2
  Add{,2..4} (4 alike) : Sum
  Add1 : Sum  Inputs=+-
  Bus Assignment : BusAssignment  AssignedSignals=slip_point.slip_angle,slip_point.theta
  Bus Assignment1 : BusAssignment  AssignedSignals=slip_point.x,slip_point.y
  Bus Selector : BusSelector  OutputSignals=slip_point.slip_angle,slip_point.w,v
  Bus Selector1 : BusSelector  OutputSignals=v
  Bus Selector2 : BusSelector  OutputSignals=img_ang
  Bus Selector3 : BusSelector  OutputSignals=img_ang,slip_point.theta
  Bus Selector4 : BusSelector  OutputSignals=slip_point.x,v,slip_point.theta
  Bus Selector5 : BusSelector  OutputSignals=slip_point.y,v,slip_point.theta
  Bus Selector6 : BusSelector  OutputSignals=slip_gain
  Constant : Constant  Value=1/dt  OutDataTypeStr=single
  Constant1 : Constant  Value=1/dt  OutDataTypeStr=single
  Constant3 : Constant  Value=0  OutDataTypeStr=single
  Cos : Trigonometry  Operator=cos
  Cos1 : Trigonometry
  Data Store Read{,1..3} (4 alike) : DataStoreRead  DataStoreName=time_step
  Data Type Conversion : DataTypeConversion  OutDataTypeStr=single
  Divide{,1..3} (4 alike) : Product  Inputs=*/
  Gain3 : Gain  Gain=dt
  Gain4 : Gain  Gain=dt
  Gain5 : Gain
  Gain6 : Gain
  Product{,1..4} (5 alike) : Product
  Scope : Scope  NumInputPorts=2
  Switch : Switch  Criteria=u2 ~= 0
  mm/s 2 m/s : Gain  Gain=0.001
  next_ego : Outport
  wires:
  ego/1 -> Bus Selector/1, Bus Assignment/1, [ego]
  Constant/1 -> Divide2/1
  Constant1/1 -> Divide3/1
  Divide3/1 -> Add/1
  Divide1/1 -> Add/2
  Add1/1 -> Divide/1
  Add/1 -> Divide/2
  Bus Selector/2 -> Add1/2  "<w>"
  Product1/1 -> Add1/1
  Divide2/1 -> Product1/1
  Bus Selector/1 -> Product1/2  "<slip_angle>"
  Bus Selector/3 -> mm/s 2 m/s/1  "<v>"
  Divide/1 -> Data Type Conversion/1
  mm/s 2 m/s/1 -> Divide1/2
  Data Type Conversion/1 -> Switch/1
  Switch/1 -> Bus Assignment/2, Add2/2
  Constant3/1 -> Switch/3
  [ego] -> Bus Selector1/1
  Bus Selector1/1 -> Switch/2  "<v>"
  Bus Selector2/1 -> Add2/1  "<img_ang>"
  [ego] -> Bus Selector2/1
  Add2/1 -> Bus Assignment/3
  Bus Selector3/1 -> Gain5/1  "<img_ang>"
  Bus Selector3/2 -> Gain6/1  "<theta>"
  Product2/1 -> Gain4/1
  Bus Selector5/1 -> Add4/1  "<y>"
  Bus Assignment/1 -> Bus Selector3/1, Bus Selector4/1, Bus Selector5/1, Bus Assignment1/1
  Bus Selector4/1 -> Add3/1  "<x>"
  Add3/1 -> Bus Assignment1/2
  Add4/1 -> Bus Assignment1/3
  Bus Selector5/3 -> Cos1/1  "<theta>"
  Bus Selector5/2 -> Product2/1  "<v>"
  Bus Selector4/2 -> Product/1  "<v>"
  Product/1 -> Gain3/1
  Cos/1 -> Product/2
  Bus Selector4/3 -> Cos/1  "<theta>"
  Cos1/1 -> Product2/2
  Bus Assignment1/1 -> next_ego/1
  Gain5/1 -> Scope/1  "ideal_angle"
  Gain6/1 -> Scope/2  "slipped_angle"
  tgt/1 -> Bus Selector6/1
  Bus Selector6/1 -> Divide1/1  "<slip_gain>"
  Data Store Read/1 -> Divide2/2
  Data Store Read1/1 -> Divide3/2
  Data Store Read2/1 -> Product3/1
  Product3/1 -> Add3/2
  Gain3/1 -> Product3/2
  Data Store Read3/1 -> Product4/1
  Product4/1 -> Add4/2
  Gain4/1 -> Product4/2

== system mpc_tgt_calc/If Action Subsystem/Subsystem2/Subsystem ==
  ego : Inport
  Add : Sum
  Bus Selector : BusSelector  OutputSignals=state,base_alpha,counter,limit_time_count
  Constant : Constant  Value=0  OutDataTypeStr=single
  Constant1 : Constant  Value=0
  Data Store Read1 : DataStoreRead  DataStoreName=time_step
  Product : Product
  Relational Operator : RelationalOperator  OutDataTypeStr=boolean  RndMeth=Simplest
  Switch : Switch  Criteria=u2 ~= 0
  Switch1 : Switch  Criteria=u2 > Threshold
  calc_neiper : Subsystem
  next_alpha : Outport
  wires:
  ego/1 -> calc_neiper/1(ego), Bus Selector/1
  Bus Selector/1 -> Switch/2  "<state>"
  Switch/1 -> next_alpha/1
  Constant/1 -> Switch/1
  Bus Selector/2 -> Product/1  "<base_alpha>"
  Product/1 -> Switch/3
  Switch1/1 -> Product/2
  calc_neiper/1(neipier) -> Switch1/3
  Relational Operator/1 -> Switch1/2
  Constant1/1 -> Switch1/1
  Bus Selector/4 -> Relational Operator/2  "<limit_time_count>"
  Data Store Read1/1 -> Add/1
  Bus Selector/3 -> Add/2  "<counter>"
  Add/1 -> Relational Operator/1

== system mpc_tgt_calc/If Action Subsystem2/Subsystem/accl ==
  alpha : Inport
  now_w : Inport  Port=2
  max_w : Inport  Port=3
  Action Port : ActionPort  ActionPortLabel=elseif(u3==0 )
  Abs : Abs
  Abs1 : Abs
  Constant : Constant  Value=0
  Constant1 : Constant  Value=0  OutDataTypeStr=int8
  Constant2 : Constant  OutDataTypeStr=int8
  Constant3 : Constant  OutDataTypeStr=single
  Constant4 : Constant  Value=2.5  OutDataTypeStr=single
  Data Type Conversion : DataTypeConversion  OutDataTypeStr=single
  Divide : Product  Inputs=*/
  Manual Switch : ManualSwitch
  Product1 : Product
  Relational Operator : RelationalOperator  Operator=<  OutDataTypeStr=boolean  RndMeth=Simplest
  Square : Math  Operator=pow  SaturateOnIntegerOverflow=on
  Subtract : Sum  Inputs=+-
  Switch : Switch  Criteria=u2 > Threshold
  Switch1 : Switch  Criteria=u2 > Threshold
  accl_out : Outport
  state_out : Outport  Port=2
  wires:
  Switch/1 -> Data Type Conversion/1
  Relational Operator/1 -> Switch1/2, Switch/2
  max_w/1 -> Divide/2, Abs1/1
  Constant/1 -> Switch/3
  alpha/1 -> [alpha], Manual Switch/1, Product1/1
  Constant1/1 -> Switch1/1
  Constant2/1 -> Switch1/3
  Constant3/1 -> Subtract/1
  Divide/1 -> Square/1
  Square/1 -> Subtract/2
  Subtract/1 -> Product1/2
  Constant4/1 -> Square/2
  Product1/1 -> Manual Switch/2
  Manual Switch/1 -> Switch/1
  now_w/1 -> Abs/1, Divide/1
  Switch1/1 -> state_out/1
  Data Type Conversion/1 -> accl_out/1
  Abs/1 -> Relational Operator/1
  Abs1/1 -> Relational Operator/2

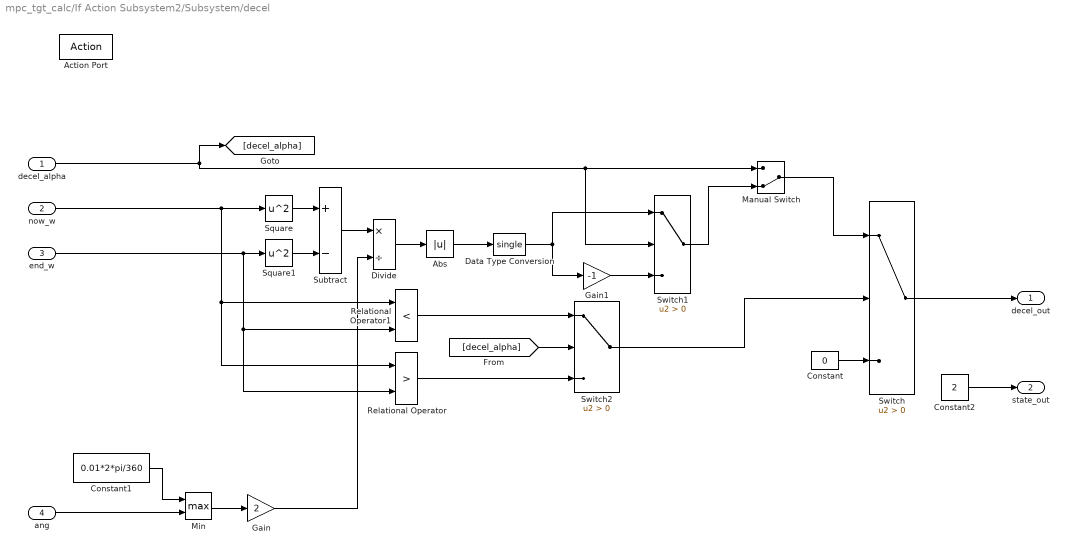
== system mpc_tgt_calc/If Action Subsystem2/Subsystem/decel ==
  decel_alpha : Inport
  now_w : Inport  Port=2
  end_w : Inport  Port=3
  ang : Inport  Port=4
  Action Port : ActionPort  ActionPortLabel=if(u3==2 | u1>=u2)
  Abs : Abs
  Constant : Constant  Value=0  OutDataTypeStr=single
  Constant1 : Constant  Value=0.01*2*pi/360
  Constant2 : Constant  Value=2  OutDataTypeStr=int8
  Data Type Conversion : DataTypeConversion  OutDataTypeStr=single
  Divide : Product  Inputs=*/
  Gain : Gain  Gain=2
  Gain1 : Gain  Gain=-1
  Manual Switch : ManualSwitch  CurrentSetting=0
  Min : MinMax  Function=max  Inputs=2
  Relational Operator : RelationalOperator  Operator=>  OutDataTypeStr=boolean  RndMeth=Simplest
  Relational Operator1 : RelationalOperator  Operator=<  OutDataTypeStr=boolean  RndMeth=Simplest
  Square : Math  Operator=square  SaturateOnIntegerOverflow=on
  Square1 : Math  Operator=square  SaturateOnIntegerOverflow=on
  Subtract : Sum  Inputs=+-
  Switch : Switch  Criteria=u2 > Threshold
  Switch1 : Switch  Criteria=u2 > Threshold
  Switch2 : Switch  Criteria=u2 > Threshold
  decel_out : Outport
  state_out : Outport  Port=2
  wires:
  Square1/1 -> Subtract/2
  Constant1/1 -> Min/1
  Min/1 -> Gain/1
  Subtract/1 -> Divide/1
  Constant/1 -> Switch/3
  Gain/1 -> Divide/2
  Divide/1 -> Abs/1
  ang/1 -> Min/2
  Square/1 -> Subtract/1
  Constant2/1 -> state_out/1
  Manual Switch/1 -> Switch/1
  decel_alpha/1 -> [decel_alpha], Switch1/2, Manual Switch/1
  end_w/1 -> Relational Operator/2, Relational Operator1/2, Square1/1
  now_w/1 -> Relational Operator/1, Relational Operator1/1, Square/1
  [decel_alpha] -> Switch2/2
  Relational Operator/1 -> Switch2/3
  Relational Operator1/1 -> Switch2/1
  Switch1/1 -> Manual Switch/2
  Abs/1 -> Data Type Conversion/1
  Gain1/1 -> Switch1/3
  Switch2/1 -> Switch/2
  Switch/1 -> decel_out/1
  Data Type Conversion/1 -> Gain1/1, Switch1/1

== system mpc_tgt_calc/If Action Subsystem2/Subsystem/keep ==
  alpha : Inport
  now_w : Inport  Port=2
  tgt_ang : Inport  Port=3
  Action Port : ActionPort  ActionPortLabel=else
  Constant : Constant  Value=0
  Constant2 : Constant  OutDataTypeStr=int8
  Data Type Conversion : DataTypeConversion  OutDataTypeStr=single
  Terminator : Terminator
  Terminator1 : Terminator
  Terminator2 : Terminator
  accl_out : Outport
  state_out : Outport  Port=2
  wires:
  Constant2/1 -> state_out/1
  Constant/1 -> Data Type Conversion/1
  Data Type Conversion/1 -> accl_out/1
  alpha/1 -> Terminator/1
  now_w/1 -> Terminator1/1
  tgt_ang/1 -> Terminator2/1

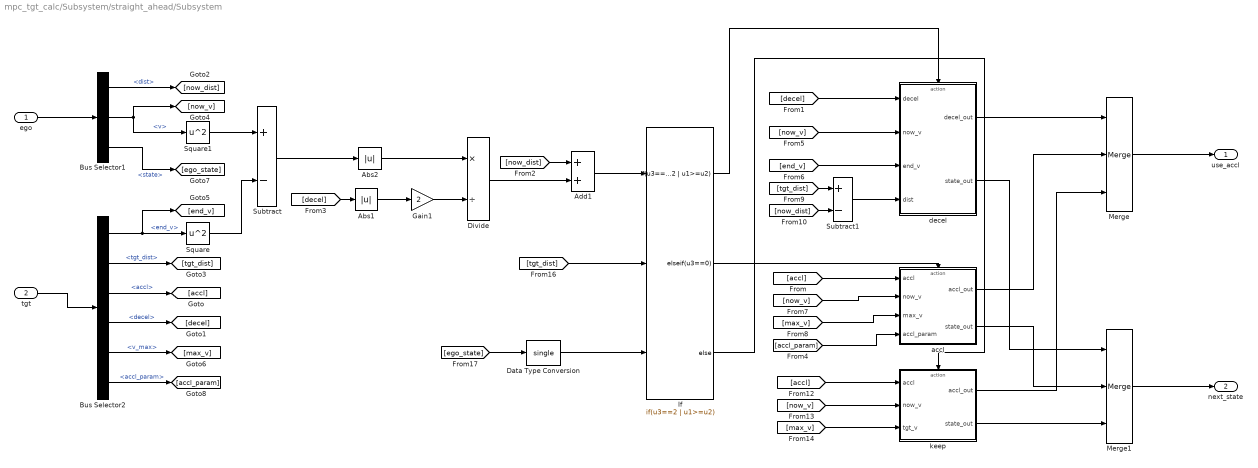
== system mpc_tgt_calc/Subsystem/straight_ahead/Subsystem ==
  ego : Inport
  tgt : Inport  Port=2
  Abs1 : Abs
  Abs2 : Abs
  Add1 : Sum
  Bus Selector1 : BusSelector  OutputSignals=dist,v,state
  Bus Selector2 : BusSelector  OutputSignals=end_v,tgt_dist,accl,decel,v_max,accl_param
  Data Type Conversion : DataTypeConversion  OutDataTypeStr=single
  Divide : Product  Inputs=*/
  Gain1 : Gain  Gain=2
  If : If  NumInputs=3  IfExpression=u3==2 | u1>=u2  ElseIfExpressions=u3==0
  Merge : Merge  Inputs=3
  Merge1 : Merge  Inputs=3
  Square : Math  Operator=square  SaturateOnIntegerOverflow=on
  Square1 : Math  Operator=square  SaturateOnIntegerOverflow=on
  Subtract : Sum  Inputs=+-
  Subtract1 : Sum  Inputs=+-
  accl : Subsystem  TreatAsAtomicUnit=on
  decel : Subsystem  TreatAsAtomicUnit=on
  keep : Subsystem  TreatAsAtomicUnit=on
  use_accl : Outport
  next_state : Outport  Port=2
  wires:
  Add1/1 -> If/1
  Gain1/1 -> Divide/2
  Square/1 -> Subtract/2
  Subtract/1 -> Abs2/1
  tgt/1 -> Bus Selector2/1
  [accl] -> accl/1(accl)
  [decel] -> decel/1(decel)
  Square1/1 -> Subtract/1
  Divide/1 -> Add1/2
  Bus Selector2/1 -> [end_v], Square/1  "<end_v>"
  ego/1 -> Bus Selector1/1
  Bus Selector1/2 -> Square1/1, [now_v]  "<v>"
  Bus Selector2/3 -> [accl]  "<accl>"
  Bus Selector2/4 -> [decel]  "<decel>"
  Bus Selector1/1 -> [now_dist]  "<dist>"
  [now_dist] -> Add1/1
  [decel] -> Abs1/1
  Abs1/1 -> Gain1/1
  Abs2/1 -> Divide/1
  Bus Selector2/2 -> [tgt_dist]  "<tgt_dist>"
  [now_v] -> decel/2(now_v)
  [end_v] -> decel/3(end_v)
  [now_v] -> accl/2(now_v)
  Bus Selector2/5 -> [max_v]  "<v_max>"
  Bus Selector1/3 -> [ego_state]  "<state>"
  Merge/1 -> use_accl/1
  [tgt_dist] -> Subtract1/1
  [now_dist] -> Subtract1/2
  Subtract1/1 -> decel/4(dist)
  [max_v] -> accl/3(max_v)
  If/3 -> keep/Action
  Merge1/1 -> next_state/1
  [accl] -> keep/1(accl)
  [now_v] -> keep/2(now_v)
  [max_v] -> keep/3(tgt_v)
  If/1 -> decel/Action
  If/2 -> accl/Action
  [tgt_dist] -> If/2
  [ego_state] -> Data Type Conversion/1
  Data Type Conversion/1 -> If/3
  keep/1(accl_out) -> Merge/3
  decel/1(decel_out) -> Merge/1
  decel/2(state_out) -> Merge1/1
  keep/2(state_out) -> Merge1/3
  accl/1(accl_out) -> Merge/2
  accl/2(state_out) -> Merge1/2
  Bus Selector2/6 -> [accl_param]  "<accl_param>"
  [accl_param] -> accl/4(accl_param)

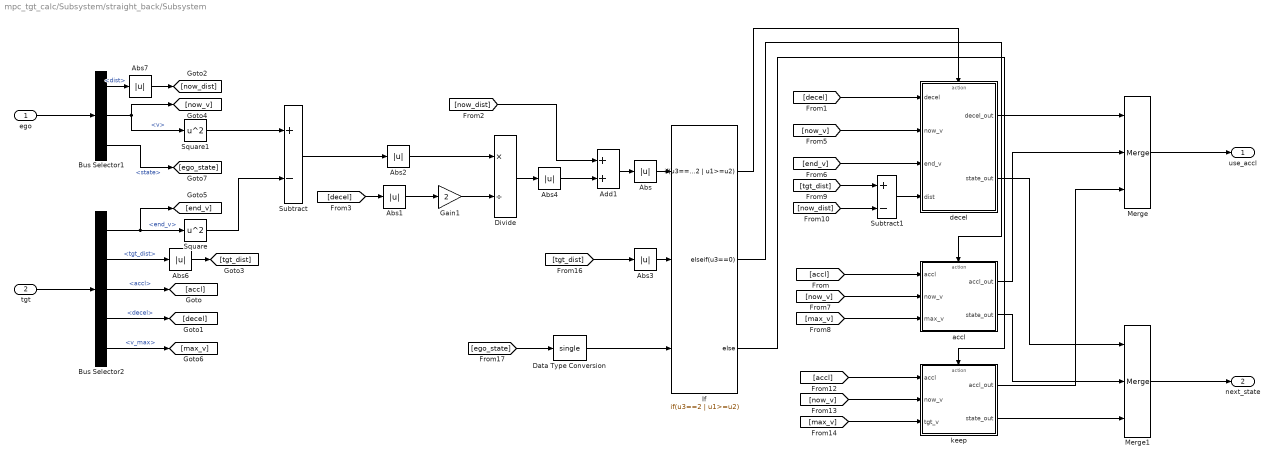
== system mpc_tgt_calc/Subsystem/straight_back/Subsystem ==
  ego : Inport
  tgt : Inport  Port=2
  Abs{,1..4,6..7} (7 alike) : Abs
  Add1 : Sum
  Bus Selector1 : BusSelector  OutputSignals=dist,v,state
  Bus Selector2 : BusSelector  OutputSignals=end_v,tgt_dist,accl,decel,v_max
  Data Type Conversion : DataTypeConversion  OutDataTypeStr=single
  Divide : Product  Inputs=*/
  Gain1 : Gain  Gain=2
  If : If  NumInputs=3  IfExpression=u3==2 | u1>=u2  ElseIfExpressions=u3==0
  Merge : Merge  Inputs=3
  Merge1 : Merge  Inputs=3
  Square : Math  Operator=square  SaturateOnIntegerOverflow=on
  Square1 : Math  Operator=square  SaturateOnIntegerOverflow=on
  Subtract : Sum  Inputs=+-
  Subtract1 : Sum  Inputs=+-
  accl : Subsystem  TreatAsAtomicUnit=on
  decel : Subsystem  TreatAsAtomicUnit=on
  keep : Subsystem  TreatAsAtomicUnit=on
  use_accl : Outport
  next_state : Outport  Port=2
  wires:
  Add1/1 -> Abs/1
  Gain1/1 -> Divide/2
  Square/1 -> Subtract/2
  Subtract/1 -> Abs2/1
  tgt/1 -> Bus Selector2/1
  [accl] -> accl/1(accl)
  [decel] -> decel/1(decel)
  Square1/1 -> Subtract/1
  Divide/1 -> Abs4/1
  Bus Selector2/1 -> [end_v], Square/1  "<end_v>"
  ego/1 -> Bus Selector1/1
  Bus Selector1/2 -> Square1/1, [now_v]  "<v>"
  Bus Selector2/3 -> [accl]  "<accl>"
  Bus Selector2/4 -> [decel]  "<decel>"
  Bus Selector1/1 -> Abs7/1  "<dist>"
  [decel] -> Abs1/1
  Abs1/1 -> Gain1/1
  Abs2/1 -> Divide/1
  Bus Selector2/2 -> Abs6/1  "<tgt_dist>"
  [now_v] -> decel/2(now_v)
  [end_v] -> decel/3(end_v)
  [now_v] -> accl/2(now_v)
  Bus Selector2/5 -> [max_v]  "<v_max>"
  Bus Selector1/3 -> [ego_state]  "<state>"
  Merge/1 -> use_accl/1
  [tgt_dist] -> Subtract1/1
  [now_dist] -> Subtract1/2
  Subtract1/1 -> decel/4(dist)
  [max_v] -> accl/3(max_v)
  If/3 -> keep/Action
  Merge1/1 -> next_state/1
  [accl] -> keep/1(accl)
  [now_v] -> keep/2(now_v)
  [max_v] -> keep/3(tgt_v)
  If/1 -> decel/Action
  If/2 -> accl/Action
  [tgt_dist] -> Abs3/1
  [ego_state] -> Data Type Conversion/1
  Data Type Conversion/1 -> If/3
  keep/1(accl_out) -> Merge/3
  decel/1(decel_out) -> Merge/1
  decel/2(state_out) -> Merge1/1
  keep/2(state_out) -> Merge1/3
  accl/1(accl_out) -> Merge/2
  accl/2(state_out) -> Merge1/2
  Abs/1 -> If/1
  Abs3/1 -> If/2
  Abs4/1 -> Add1/2
  [now_dist] -> Add1/1
  Abs6/1 -> [tgt_dist]
  Abs7/1 -> [now_dist]

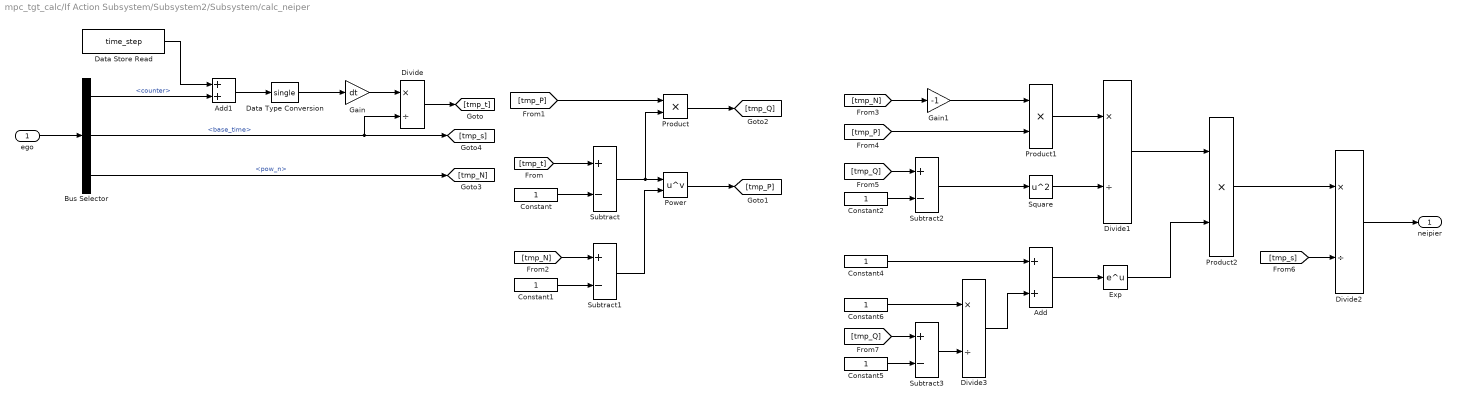
== system mpc_tgt_calc/If Action Subsystem/Subsystem2/Subsystem/calc_neiper ==
  ego : Inport
  Add : Sum
  Add1 : Sum
  Bus Selector : BusSelector  OutputSignals=counter,base_time,pow_n
  Constant{,1..2,4..6} (6 alike) : Constant  OutDataTypeStr=single
  Data Store Read : DataStoreRead  DataStoreName=time_step
  Data Type Conversion : DataTypeConversion  OutDataTypeStr=single
  Divide{,1..3} (4 alike) : Product  Inputs=*/
  Exp : Math  SaturateOnIntegerOverflow=on
  Gain : Gain  Gain=dt
  Gain1 : Gain  Gain=-1
  Power : Math  Operator=pow  SaturateOnIntegerOverflow=on
  Product : Product
  Product1 : Product
  Product2 : Product
  Square : Math  Operator=square  SaturateOnIntegerOverflow=on
  Subtract{,1..3} (4 alike) : Sum  Inputs=+-
  neipier : Outport
  wires:
  ego/1 -> Bus Selector/1
  Gain/1 -> Divide/1
  Bus Selector/2 -> Divide/2, [tmp_s]  "<base_time>"
  Divide/1 -> [tmp_t]
  [tmp_t] -> Subtract/1
  Constant/1 -> Subtract/2
  Subtract/1 -> Power/1, Product/2
  Subtract1/1 -> Power/2
  Constant1/1 -> Subtract1/2
  Power/1 -> [tmp_P]
  [tmp_P] -> Product/1
  Product/1 -> [tmp_Q]
  Bus Selector/3 -> [tmp_N]  "<pow_n>"
  [tmp_N] -> Subtract1/1
  [tmp_N] -> Gain1/1
  Gain1/1 -> Product1/1
  [tmp_P] -> Product1/2
  Product1/1 -> Divide1/1
  [tmp_Q] -> Subtract2/1
  Constant2/1 -> Subtract2/2
  Subtract2/1 -> Square/1
  Square/1 -> Divide1/2
  Divide1/1 -> Product2/1
  Product2/1 -> Divide2/1
  [tmp_s] -> Divide2/2
  Constant4/1 -> Add/1
  [tmp_Q] -> Subtract3/1
  Constant5/1 -> Subtract3/2
  Divide3/1 -> Add/2
  Subtract3/1 -> Divide3/2
  Constant6/1 -> Divide3/1
  Add/1 -> Exp/1
  Exp/1 -> Product2/2
  Divide2/1 -> neipier/1
  Bus Selector/1 -> Add1/2  "<counter>"
  Data Type Conversion/1 -> Gain/1
  Data Store Read/1 -> Add1/1
  Add1/1 -> Data Type Conversion/1

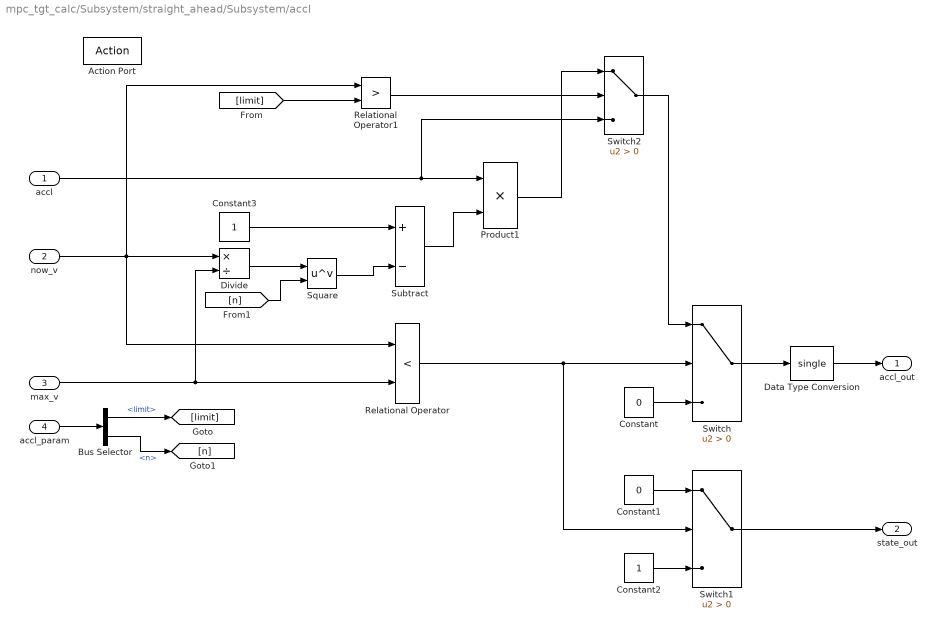
== system mpc_tgt_calc/Subsystem/straight_ahead/Subsystem/accl ==
  accl : Inport
  now_v : Inport  Port=2
  max_v : Inport  Port=3
  accl_param : Inport  Port=4
  Action Port : ActionPort  ActionPortLabel=elseif(u3==0 )
  Bus Selector : BusSelector  OutputSignals=limit,n
  Constant : Constant  Value=0
  Constant1 : Constant  Value=0  OutDataTypeStr=int8
  Constant2 : Constant  OutDataTypeStr=int8
  Constant3 : Constant  OutDataTypeStr=single
  Data Type Conversion : DataTypeConversion  OutDataTypeStr=single
  Divide : Product  Inputs=*/
  Product1 : Product
  Relational Operator : RelationalOperator  Operator=<  OutDataTypeStr=boolean  RndMeth=Simplest
  Relational Operator1 : RelationalOperator  Operator=>  OutDataTypeStr=boolean  RndMeth=Simplest
  Square : Math  Operator=pow  SaturateOnIntegerOverflow=on
  Subtract : Sum  Inputs=+-
  Switch : Switch  Criteria=u2 > Threshold
  Switch1 : Switch  Criteria=u2 > Threshold
  Switch2 : Switch  Criteria=u2 > Threshold
  accl_out : Outport
  state_out : Outport  Port=2
  wires:
  Switch/1 -> Data Type Conversion/1
  now_v/1 -> Relational Operator1/1, Relational Operator/1, Divide/1
  Relational Operator/1 -> Switch/2, Switch1/2
  max_v/1 -> Relational Operator/2, Divide/2
  Constant/1 -> Switch/3
  Data Type Conversion/1 -> accl_out/1
  accl/1 -> Switch2/3, Product1/1
  Switch1/1 -> state_out/1
  Constant1/1 -> Switch1/1
  Constant2/1 -> Switch1/3
  Constant3/1 -> Subtract/1
  Divide/1 -> Square/1
  Square/1 -> Subtract/2
  Subtract/1 -> Product1/2
  [n] -> Square/2
  Switch2/1 -> Switch/1
  Product1/1 -> Switch2/1
  Relational Operator1/1 -> Switch2/2
  accl_param/1 -> Bus Selector/1
  Bus Selector/1 -> [limit]  "<limit>"
  Bus Selector/2 -> [n]  "<n>"
  [limit] -> Relational Operator1/2

== system mpc_tgt_calc/Subsystem/straight_ahead/Subsystem/decel ==
  decel : Inport
  now_v : Inport  Port=2
  end_v : Inport  Port=3
  dist : Inport  Port=4
  Action Port : ActionPort  ActionPortLabel=if(u3==2 | u1>=u2)
  Abs : Abs
  Constant : Constant  Value=0
  Constant1 : Constant  Value=0.01
  Constant2 : Constant  Value=2  OutDataTypeStr=int8
  Data Type Conversion : DataTypeConversion  OutDataTypeStr=single
  Divide : Product  Inputs=*/
  Gain : Gain  Gain=2
  Gain1 : Gain  Gain=-1
  Manual Switch : ManualSwitch  CurrentSetting=0
  Min : MinMax  Function=max  Inputs=2
  Relational Operator : RelationalOperator  Operator=>  OutDataTypeStr=boolean  RndMeth=Simplest
  Square : Math  Operator=square  SaturateOnIntegerOverflow=on
  Square1 : Math  Operator=square  SaturateOnIntegerOverflow=on
  Subtract : Sum  Inputs=+-
  Switch : Switch  Criteria=u2 > Threshold
  decel_out : Outport
  state_out : Outport  Port=2
  wires:
  Square1/1 -> Subtract/2
  Constant1/1 -> Min/1
  Abs/1 -> Gain1/1
  Gain1/1 -> Manual Switch/2
  Min/1 -> Gain/1
  Switch/1 -> Data Type Conversion/1
  Relational Operator/1 -> Switch/2
  Subtract/1 -> Divide/1
  Constant/1 -> Switch/3
  Gain/1 -> Divide/2
  Divide/1 -> Abs/1
  dist/1 -> Min/2
  Square/1 -> Subtract/1
  Constant2/1 -> state_out/1
  Data Type Conversion/1 -> decel_out/1
  Manual Switch/1 -> Switch/1
  decel/1 -> Manual Switch/1
  end_v/1 -> Relational Operator/2, Square1/1
  now_v/1 -> Relational Operator/1, Square/1

== system mpc_tgt_calc/Subsystem/straight_ahead/Subsystem/keep ==
  accl : Inport
  now_v : Inport  Port=2
  tgt_v : Inport  Port=3
  Action Port : ActionPort  ActionPortLabel=else
  Constant : Constant  Value=0
  Constant2 : Constant  OutDataTypeStr=int8
  Data Type Conversion : DataTypeConversion  OutDataTypeStr=single
  Terminator : Terminator
  Terminator1 : Terminator
  Terminator2 : Terminator
  accl_out : Outport
  state_out : Outport  Port=2
  wires:
  Constant2/1 -> state_out/1
  Constant/1 -> Data Type Conversion/1
  Data Type Conversion/1 -> accl_out/1
  accl/1 -> Terminator/1
  now_v/1 -> Terminator1/1
  tgt_v/1 -> Terminator2/1

== system mpc_tgt_calc/Subsystem/straight_back/Subsystem/accl ==
  accl : Inport
  now_v : Inport  Port=2
  max_v : Inport  Port=3
  Action Port : ActionPort  ActionPortLabel=elseif(u3==0 )
  Constant : Constant  Value=0
  Constant1 : Constant  Value=0  OutDataTypeStr=int8
  Constant2 : Constant  OutDataTypeStr=int8
  Constant3 : Constant  OutDataTypeStr=single
  Constant4 : Constant  Value=2.5  OutDataTypeStr=single
  Data Type Conversion : DataTypeConversion  OutDataTypeStr=single
  Divide : Product  Inputs=*/
  Manual Switch : ManualSwitch  CurrentSetting=0
  Product1 : Product
  Relational Operator : RelationalOperator  Operator=>  OutDataTypeStr=boolean  RndMeth=Simplest
  Square : Math  Operator=pow  SaturateOnIntegerOverflow=on
  Subtract : Sum  Inputs=+-
  Switch : Switch  Criteria=u2 > Threshold
  Switch1 : Switch  Criteria=u2 > Threshold
  accl_out : Outport
  state_out : Outport  Port=2
  wires:
  Switch/1 -> Data Type Conversion/1
  now_v/1 -> Relational Operator/1, Divide/1
  Relational Operator/1 -> Switch/2, Switch1/2
  max_v/1 -> Relational Operator/2, Divide/2
  Constant/1 -> Switch/3
  Data Type Conversion/1 -> accl_out/1
  accl/1 -> Manual Switch/1, Product1/1
  Switch1/1 -> state_out/1
  Constant1/1 -> Switch1/1
  Constant2/1 -> Switch1/3
  Constant3/1 -> Subtract/1
  Divide/1 -> Square/1
  Square/1 -> Subtract/2
  Subtract/1 -> Product1/2
  Constant4/1 -> Square/2
  Manual Switch/1 -> Switch/1
  Product1/1 -> Manual Switch/2

== system mpc_tgt_calc/Subsystem/straight_back/Subsystem/decel ==
  decel : Inport
  now_v : Inport  Port=2
  end_v : Inport  Port=3
  dist : Inport  Port=4
  Action Port : ActionPort  ActionPortLabel=if(u3==2 | u1>=u2)
  Abs : Abs
  Constant : Constant  Value=0
  Constant1 : Constant  Value=0.01
  Constant2 : Constant  Value=2  OutDataTypeStr=int8
  Data Type Conversion : DataTypeConversion  OutDataTypeStr=single
  Divide : Product  Inputs=*/
  Gain : Gain  Gain=2
  Gain1 : Gain
  Manual Switch : ManualSwitch  CurrentSetting=0
  Min : MinMax  Function=max  Inputs=2
  Relational Operator : RelationalOperator  Operator=<  OutDataTypeStr=boolean  RndMeth=Simplest
  Square : Math  Operator=square  SaturateOnIntegerOverflow=on
  Square1 : Math  Operator=square  SaturateOnIntegerOverflow=on
  Subtract : Sum  Inputs=+-
  Switch : Switch  Criteria=u2 > Threshold
  decel_out : Outport
  state_out : Outport  Port=2
  wires:
  Square1/1 -> Subtract/2
  Constant1/1 -> Min/1
  Abs/1 -> Gain1/1
  Gain1/1 -> Manual Switch/2
  Min/1 -> Gain/1
  Switch/1 -> Data Type Conversion/1
  Relational Operator/1 -> Switch/2
  Subtract/1 -> Divide/1
  Constant/1 -> Switch/3
  Gain/1 -> Divide/2
  Divide/1 -> Abs/1
  dist/1 -> Min/2
  Square/1 -> Subtract/1
  Constant2/1 -> state_out/1
  Data Type Conversion/1 -> decel_out/1
  Manual Switch/1 -> Switch/1
  decel/1 -> Manual Switch/1
  end_v/1 -> Relational Operator/2, Square1/1
  now_v/1 -> Relational Operator/1, Square/1

== system mpc_tgt_calc/Subsystem/straight_back/Subsystem/keep ==
  accl : Inport
  now_v : Inport  Port=2
  tgt_v : Inport  Port=3
  Action Port : ActionPort  ActionPortLabel=else
  Constant : Constant  Value=0
  Constant2 : Constant  OutDataTypeStr=int8
  Data Type Conversion : DataTypeConversion  OutDataTypeStr=single
  Terminator : Terminator
  Terminator1 : Terminator
  Terminator2 : Terminator
  accl_out : Outport
  state_out : Outport  Port=2
  wires:
  Constant2/1 -> state_out/1
  Constant/1 -> Data Type Conversion/1
  Data Type Conversion/1 -> accl_out/1
  accl/1 -> Terminator/1
  now_v/1 -> Terminator1/1
  tgt_v/1 -> Terminator2/1

== matlab function mpc_tgt_calc/kanayama_ctrl_method1/MATLAB Function ==
  data: x output; ego input Bus: t_ego; y output; theta output; tgt input Bus: t_tgt
function [x, y,theta]  = detect_trj_point_impl(ego, tgt)
    [x, y, ~, theta, ~] = detect_trj_point(ego, tgt);
end
